simulink model "loop_shaping"  (R2015a)
settings: Solver=ode45  StartTime=0.0  StopTime=10.0  RelTol=1e-3
InitFcn:
  | param
values from neighbouring files (symbols this model uses):
  Ch = 9    [param.m]
  gain_c = 1    [param.m]
  gain_p = -0.03    [param.m]
  Ke = -1.0000e+05    (= -100000)    [param.m]
  Kh = 625    [param.m]
  L = 0.0220    (= 0.022)    [param.m]
  M = 1.35    [param.m]
  pole1 = -100    [param.m]
  R = 1.3    [param.m]
  zero1 = -5+22i    [param.m]
  zero2 = -5-22i    [param.m]
libraries: simulink x1
settings Model: CovModelRefEnable=off  Creator=gsavaia  LastModifiedBy=GSavaia
settings DataIOCC: SaveFormat=Dataset
settings HardwareCC: ProdBitPerPointer=64  ProdLargestAtomicFloat=Float  ProdIntDivRoundTo=Zero  ProdEndianess=LittleEndian  ProdHWDeviceType=Specified
settings GRTTargetCC: GeneratePreprocessorConditionals=Use local settings

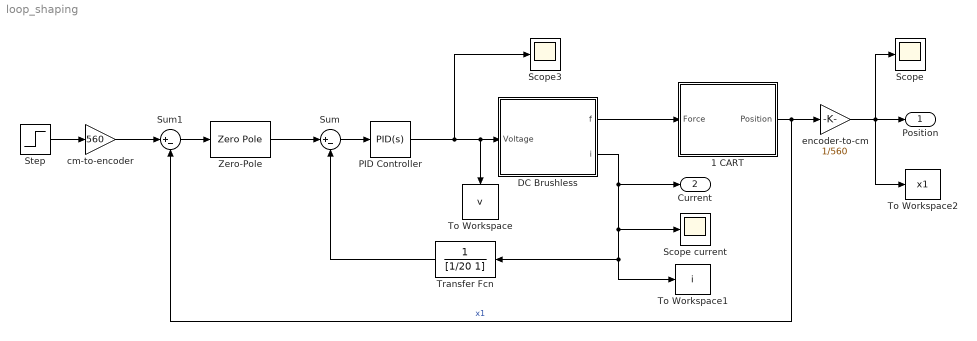
== system loop_shaping ==
  1 CART : Subsystem
  DC Brushless : Subsystem
  PID Controller : simulink/Continuous/PID Controller  Controller=PID  TimeDomain=Continuous-time  SampleTime=-1  IntegratorMethod=Forward Euler  FilterMethod=Forward Euler  Form=Parallel  UseFilter=on  ControllerParametersSource=internal  P=gain_c  I=0  D=0  N=100  InitialConditionSource=internal  InitialConditionForIntegrator=0  InitialConditionForFilter=0  ExternalReset=none  LimitOutput=off  UpperSaturationLimit=inf  LowerSaturationLimit=-inf  LinearizeAsGain=on  AntiWindupMode=none  Kb=1  TrackingMode=off  Kt=1  PParamMin=[]  PParamMax=[]  IParamMin=[]  IParamMax=[]  DParamMin=[]  DParamMax=[]  NParamMin=[]  NParamMax=[]  KbParamMin=[]  KbParamMax=[]  KtParamMin=[]  KtParamMax=[]  POutMin=[]  POutMax=[]  IOutMin=[]  IOutMax=[]  DOutMin=[]  DOutMax=[]  NOutMin=[]  NOutMax=[]  KbOutMin=[]  KbOutMax=[]  KtOutMin=[]  KtOutMax=[]  IntegratorOutMin=[]  IntegratorOutMax=[]  FilterOutMin=[]  FilterOutMax=[]  SumOutMin=[]  SumOutMax=[]  SumI1OutMin=[]  SumI1OutMax=[]  SumI2OutMin=[]  SumI2OutMax=[]  SumI3OutMin=[]  SumI3OutMax=[]  SumDOutMin=[]  SumDOutMax=[]  SaturationOutMin=[]  SaturationOutMax=[]  IntegratorContinuousStateAttributes=''  IntegratorStateMustResolveToSignalObject=off  IntegratorRTWStateStorageClass=Auto  FilterContinuousStateAttributes=''  FilterStateMustResolveToSignalObject=off  FilterRTWStateStorageClass=Auto  DifferentiatorICPrevScaledInput=0  DifferentiatorOutMin=[]  DifferentiatorOutMax=[]
  Scope : Scope
      settings: YMin=-0.01  YMax=0.01
  Scope current : Scope
      settings: YMin=-0.01  YMax=0.01
  Scope3 : Scope
      settings: TimeRange=10  YMin=0  YMax=1000  SaveName=ScopeData4
  Step : Step  SampleTime=0
  Sum : Sum  Inputs=|+-
  Sum1 : Sum  Inputs=|+-
  To Workspace : ToWorkspace  VariableName=v  SaveFormat=Timeseries  SampleTime=-1
  To Workspace1 : ToWorkspace  VariableName=i  SaveFormat=Timeseries  SampleTime=-1
  To Workspace2 : ToWorkspace  VariableName=x1  SaveFormat=Timeseries  SampleTime=-1
  Transfer Fcn : TransferFcn  Denominator=[1/20 1]
  Zero-Pole : ZeroPole  Zeros=[zero1, zero2]  Poles=[0, pole1]  Gain=gain_p
  cm-to-encoder : Gain  Gain=560
  encoder-to-cm : Gain  Gain=1/560
  Position : Outport
  Current : Outport  Port=2
  wires:
  DC Brushless/1("f ") -> 1 CART/1(Force)
  1 CART/1(Position) -> encoder-to-cm/1, Sum1/2  "x1"
  PID Controller/1 -> To Workspace/1, DC Brushless/1("Voltage "), Scope3/1
  DC Brushless/2(i) -> Current/1, Transfer Fcn/1, To Workspace1/1, Scope current/1
  Sum/1 -> PID Controller/1
  Sum1/1 -> Zero-Pole/1
  Zero-Pole/1 -> Sum/1
  Transfer Fcn/1 -> Sum/2
  cm-to-encoder/1 -> Sum1/1
  Step/1 -> cm-to-encoder/1
  encoder-to-cm/1 -> Position/1, To Workspace2/1, Scope/1

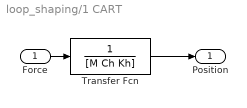
== system loop_shaping/1 CART ==
  Force : Inport
  Transfer Fcn : TransferFcn  Denominator=[M Ch Kh]
  Position : Outport
  wires:
  Force/1 -> Transfer Fcn/1
  Transfer Fcn/1 -> Position/1

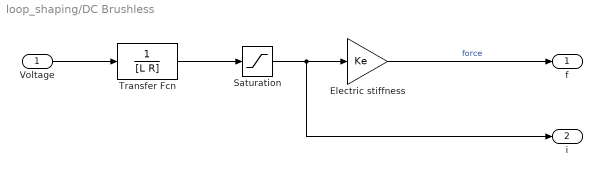
== system loop_shaping/DC Brushless ==
  "Voltage " : Inport
  Electric stiffness : Gain  Gain=Ke
  Saturation : Saturate  UpperLimit=4.2  LowerLimit=-10
  Transfer Fcn : TransferFcn  Denominator=[L R]
  "f " : Outport
  i : Outport  Port=2
  wires:
  "Voltage "/1 -> Transfer Fcn/1
  Electric stiffness/1 -> "f "/1  "force"
  Transfer Fcn/1 -> Saturation/1
  Saturation/1 -> i/1, Electric stiffness/1
